simulink model "lab4pt2"  (Simulink 8.0)
settings: Solver=ode45  StartTime=0.0  StopTime=10.0  RelTol=1e-3
libraries: simulink_extras x1
settings Model: Creator=Admin  LastModifiedBy=vukovic8
settings DataIOCC: SignalLoggingSaveFormat=ModelDataLogs
settings OptimizationCC: ExpressionDepthLimit=128
settings DebuggingCC: MultiTaskDSMMsg=warning  MultiTaskCondExecSysMsg=none  StrictBusMsg=None
settings RTWCC: IncludeERTFirstTime=on
settings CodeAppCC: CustomSymbolStrType=$N$R$M_T  InternalIdentifier=Shortened

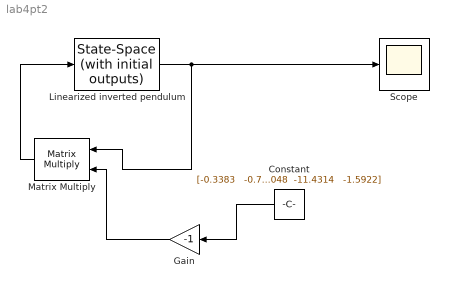
== system lab4pt2 ==
  Constant : Constant  Value="[-0.3383   -0.7048  -11.4314   -1.5922]"
  Gain : Gain  Gain=-1
  Linearized inverted pendulum : simulink_extras/Additional Linear/State-Space (with initial outputs)  A=[0,1,0,0; 0,0,-4.5138,0; 0,0,0,1; 0,0,47.1744,0]  B=[0; 2.1978; 0; -7.2535]  C=eye(4)  D=[0;0;0;0]  U0=1  Y0=[0; 0; 0.035; 0.01]
  Matrix Multiply : Product  Multiplication=Matrix(*)
  Scope : Scope
      settings: ShowLegends=on
  wires:
  Linearized inverted pendulum/1 -> Scope/1, Matrix Multiply/1
  Matrix Multiply/1 -> Linearized inverted pendulum/1
  Constant/1 -> Gain/1
  Gain/1 -> Matrix Multiply/2
